simulink model "prob4_MBD"  (R2020b)
settings: Solver=VariableStepAuto  StartTime=0.0  StopTime=10.0  RelTol=1e-3
settings Model: Creator=Ani  LastModifiedBy=Ani

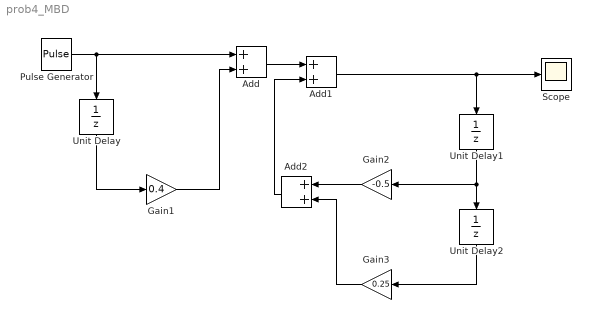
== system prob4_MBD ==
  Add : Sum
  Add1 : Sum
  Add2 : Sum
  Gain1 : Gain  Gain=0.4
  Gain2 : Gain  Gain=-0.5
  Gain3 : Gain  Gain=0.25
  Pulse Generator : DiscretePulseGenerator  PulseType=Time based  Period=10  PulseWidth=5
  Scope : Scope
  Unit Delay : UnitDelay  SampleTime=-1  HasFrameUpgradeWarning=on
  Unit Delay1 : UnitDelay  SampleTime=-1  HasFrameUpgradeWarning=on
  Unit Delay2 : UnitDelay  SampleTime=-1  HasFrameUpgradeWarning=on
  wires:
  Gain2/1 -> Add2/1
  Gain3/1 -> Add2/2
  Add1/1 -> Scope/1, Unit Delay1/1
  Add2/1 -> Add1/2
  Gain1/1 -> Add/2
  Unit Delay1/1 -> Gain2/1, Unit Delay2/1
  Unit Delay/1 -> Gain1/1
  Pulse Generator/1 -> Add/1, Unit Delay/1
  Unit Delay2/1 -> Gain3/1
  Add/1 -> Add1/1
